simulink model "QUESTION3_1_OCF"  (R2021a)
settings: Solver=VariableStepAuto  StartTime=0.0  StopTime=10.0  RelTol=1e-3
settings Model: Creator=user  LastModifiedBy=user

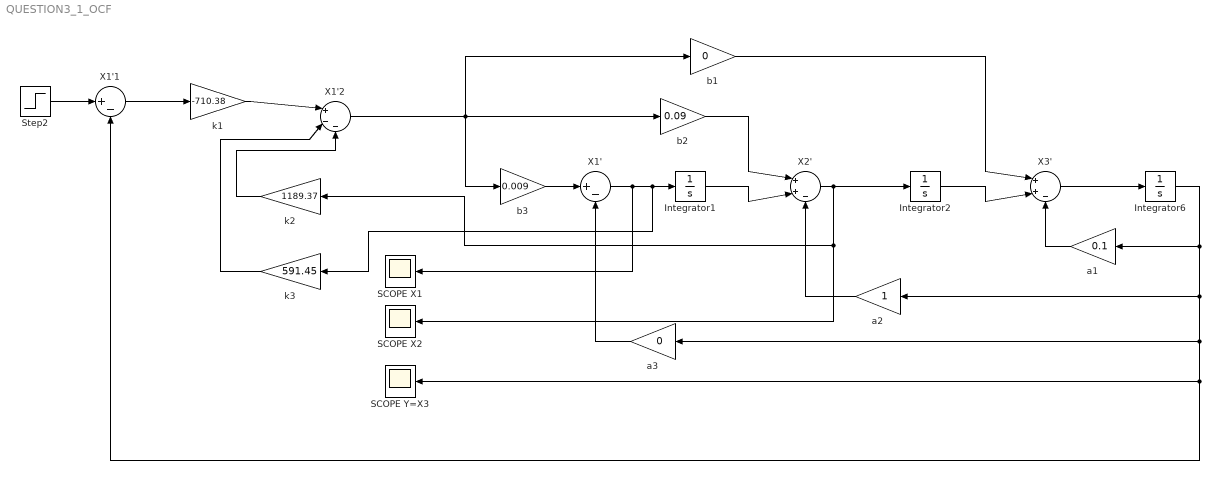
== system QUESTION3_1_OCF ==
  Integrator1 : Integrator
  Integrator2 : Integrator
  Integrator6 : Integrator
  SCOPE X1 : Scope
  SCOPE X2 : Scope
  SCOPE Y=X3 : Scope
  Step2 : Step  SampleTime=0
  X1' : Sum  Inputs=|+-
  X1'1 : Sum  Inputs=|+-
  X1'2 : Sum  Inputs=|+--
  X2' : Sum  Inputs=|++-
  X3' : Sum  Inputs=|++-
  a1 : Gain  Gain=0.1
  a2 : Gain
  a3 : Gain  Gain=0
  b1 : Gain  Gain=0
  b2 : Gain  Gain=0.09
  b3 : Gain  Gain=0.009
  k1 : Gain  Gain=-710.38
  k2 : Gain  Gain=1189.37
  k3 : Gain  Gain=591.45
  wires:
  a3/1 -> X1'/2
  Integrator6/1 -> a1/1, a2/1, SCOPE Y=X3/1, X1'1/2, a3/1
  X1'/1 -> SCOPE X1/1, k3/1, Integrator1/1
  b3/1 -> X1'/1
  X2'/1 -> Integrator2/1, SCOPE X2/1, k2/1
  Integrator2/1 -> X3'/2
  X3'/1 -> Integrator6/1
  Integrator1/1 -> X2'/2
  b2/1 -> X2'/1
  b1/1 -> X3'/1
  a1/1 -> X3'/3
  a2/1 -> X2'/3
  Step2/1 -> X1'1/1
  X1'1/1 -> k1/1
  k1/1 -> X1'2/1
  X1'2/1 -> b2/1, b1/1, b3/1
  k2/1 -> X1'2/3
  k3/1 -> X1'2/2
